simulink model "exercise5q1"  (R2023b)
settings: Solver=ode1  StartTime=0.0  StopTime=10.0  FixedStep=1/1000  RelTol=1e-3
undefined symbols (not defined in the file or in its folder): H
settings Model: Creator=bengo  LastModifiedBy=bengo

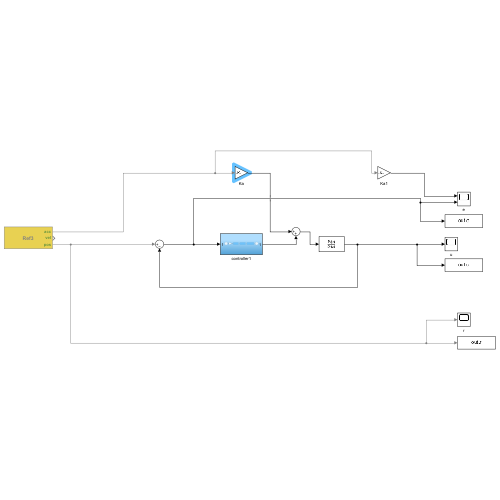
[thumbnail: Simulink's stored preview of the top-level diagram]
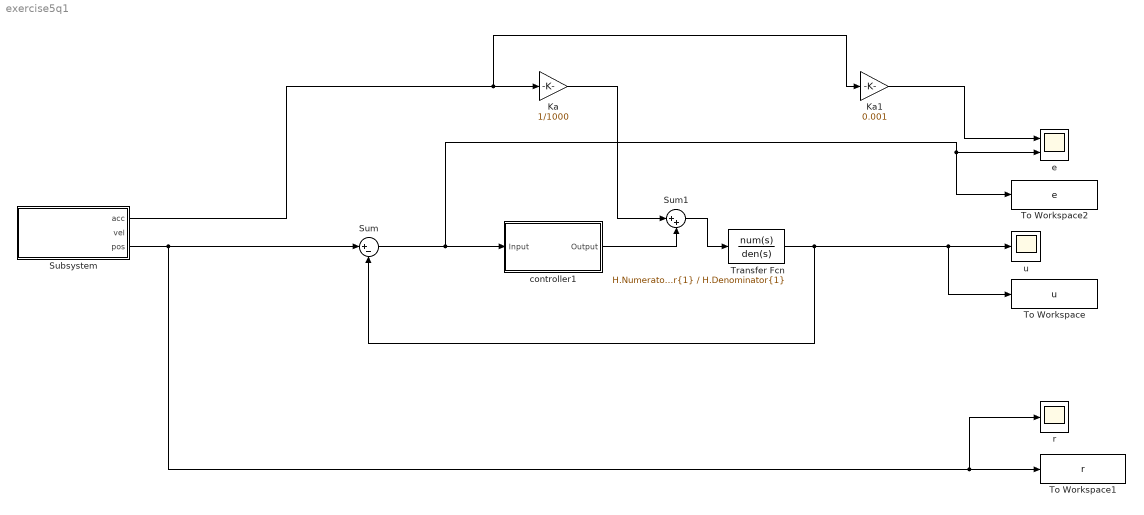
== system exercise5q1 ==
  Ka : Gain  Gain=1/1000
  Ka1 : Gain  Gain=0.001
  Subsystem : Subsystem  mask(Ref3){}
      settings: OpenFcn=r3g_main
      mask Display: disp('Ref3');
  Sum : Sum  Inputs=|+-
  Sum1 : Sum  Inputs=|++
  To Workspace : ToWorkspace  VariableName=u  SaveFormat=Timeseries  SampleTime=-1
  To Workspace1 : ToWorkspace  VariableName=r  SaveFormat=Timeseries  SampleTime=-1
  To Workspace2 : ToWorkspace  VariableName=e  SaveFormat=Timeseries  SampleTime=-1
  Transfer Fcn : TransferFcn  Numerator=H.Numerator{1}  Denominator=H.Denominator{1}
  controller1 : Subsystem
  e : Scope  NumInputPorts=2
  r : Scope
  u : Scope
  wires:
  controller1/1(Output) -> Sum1/2
  Sum/1 -> controller1/1(Input), To Workspace2/1, e/2
  Subsystem/3(pos) -> r/1, To Workspace1/1, Sum/1
  Transfer Fcn/1 -> To Workspace/1, u/1, Sum/2
  Subsystem/1(acc) -> Ka1/1, Ka/1
  Sum1/1 -> Transfer Fcn/1
  Ka/1 -> Sum1/1
  Ka1/1 -> e/1

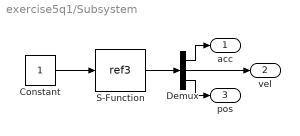
== system exercise5q1/Subsystem ==
  Constant : Constant
  Demux : Demux  Outputs=3
      settings: DisplayOption=none
  S-Function : S-Function  FunctionName=ref3  Parameters=ref_part  SFunctionDeploymentMode=off  EnableBusSupport=off
      settings: OpenFcn=global ref_part; r3g_main
  acc : Outport
  vel : Outport  Port=2
  pos : Outport  Port=3
  wires:
  Constant/1 -> S-Function/1
  S-Function/1 -> Demux/1
  Demux/1 -> acc/1
  Demux/2 -> vel/1
  Demux/3 -> pos/1

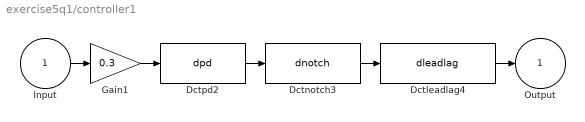
== system exercise5q1/controller1 ==
  Input : Inport
  Dctleadlag4 : S-Function  FunctionName=dleadlag  Parameters=f_num, f_den, 0.001  SFunctionDeploymentMode=off  EnableBusSupport=off  mask(dctools){f_num=3.3333, f_den=30}
      mask prompts: f_num "Zero [Hz]"; f_den "Pole [Hz]"
      mask help: This block implements a discrete time leadlag filter.
      mask Display: disp('DCT leadlag')
  Dctnotch3 : S-Function  FunctionName=dnotch  Parameters=f_num, b_num, f_den, b_den, 0.001  SFunctionDeploymentMode=off  EnableBusSupport=off  mask(dctools){f_num=9, b_num=0.2, f_den=20, b_den=0.9}
      mask prompts: f_num "Zero [Hz]"; b_num "Damping zero [-]"; f_den "Pole [Hz]"; b_den "Damping pole [-]"
      mask help: This block implements a dicrete time 2nd order notch filter.
      mask Display: disp('DCT notch')
  Dctpd2 : S-Function  FunctionName=dpd  Parameters=kp, kv, 0.001  SFunctionDeploymentMode=off  EnableBusSupport=off  mask(dctools){kp=1, kv=0.1}
      mask help: This block implements a discrete time pd filter.
      mask Display: disp('DCT pd')
  Gain1 : Gain  Gain=0.3
  Output : Outport
  wires:
  Input/1 -> Gain1/1
  Gain1/1 -> Dctpd2/1
  Dctpd2/1 -> Dctnotch3/1
  Dctnotch3/1 -> Dctleadlag4/1
  Dctleadlag4/1 -> Output/1
